simulink model "Test_model"  (R2021a)
settings: Solver=VariableStepAuto  StartTime=0.0  StopTime=5  FixedStep=0.1  RelTol=1e-3
values from neighbouring files (symbols this model uses):
  model = robotics.core.internal.navigation.ModelFactory.getMotionModel(obj.ModelType, obj.DataType)    [StateVector2StructModForEach.m]
  N_j = nonzeros(N_j)    [coordination_linear.m]    (also in init_traj.m = constraints.N_j)
  r = constraints.r    [init_traj.m]
  x0 = constraints.x0    [init_traj.m]
undefined symbols (not defined in the file or in its folder): ADMM_vec, constraints_struct, Objective
libraries: dspswit3 x1, uavGuidanceForEachMod x1, dspindex x1
settings Model: Creator=worc4873  LastModifiedBy=worc4873
settings DebuggingCC: ReadBeforeWriteMsg=DisableAll  WriteAfterWriteMsg=DisableAll  WriteAfterReadMsg=DisableAll  MultiTaskDSMMsg=none
settings ModelReferenceCC: UpdateModelReferenceTargets=IfOutOfDate
settings SFSimCC: SFSimEcho=off

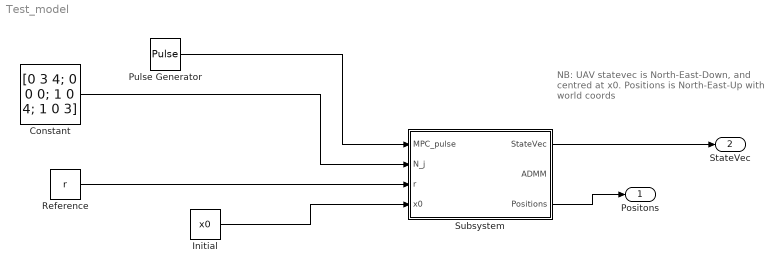
== system Test_model ==
  note: NB: UAV statevec is North-East-Down, and centred at x0. Positions is North-East-Up with world coords
  Constant : Constant  Value=[0 3 4; 0 0 0; 1 0 4; 1 0 3]
  Initial : Constant  Value=x0
  Pulse Generator : DiscretePulseGenerator  Period=10  PhaseDelay=1  SampleTime=0.1
  Reference : Constant  Value=r
  Subsystem : Subsystem
  Positons : Outport
  StateVec : Outport  Port=2
  wires:
  Pulse Generator/1 -> Subsystem/1(MPC_pulse)
  Constant/1 -> Subsystem/2(N_j)
  Reference/1 -> Subsystem/3(r)
  Initial/1 -> Subsystem/4(x0)
  Subsystem/1(StateVec) -> StateVec/1
  Subsystem/3(Positions) -> Positons/1

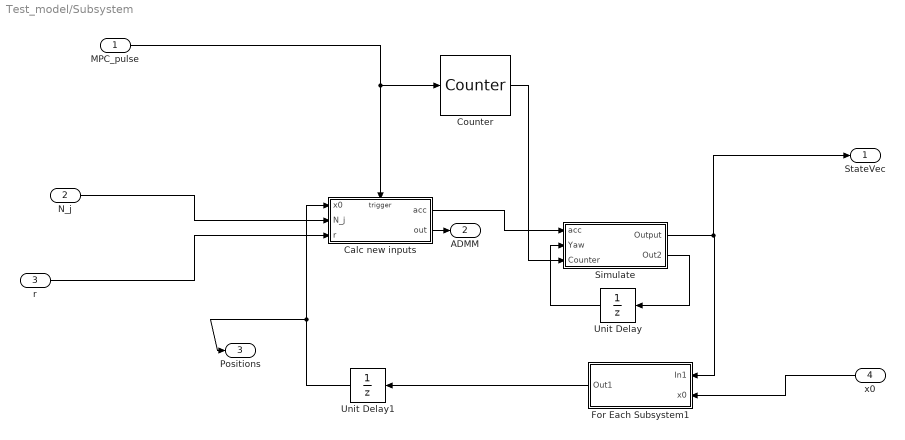
== system Test_model/Subsystem ==
  MPC_pulse : Inport
  N_j : Inport  Port=2
  r : Inport  Port=3
  x0 : Inport  Port=4
  Calc new inputs : Subsystem  TreatAsAtomicUnit=on
  Counter : dspswit3/Counter  Direction=Up  CountEvent=Free running  CounterSize=User defined  MaxCount=30  InitialCount=0  Output=Count  HitValue=32  ResetInput=on  SamplesPerFrame=1  Ts=0.1  CntDtype=double  HitDtype=Logical
  For Each Subsystem1 : Subsystem  TreatAsAtomicUnit=on
  Simulate : Subsystem  TreatAsAtomicUnit=on
  Unit Delay : UnitDelay  SampleTime=-1  HasFrameUpgradeWarning=on
  Unit Delay1 : UnitDelay  InitialCondition=x0  SampleTime=-1  HasFrameUpgradeWarning=on
  StateVec : Outport
  ADMM : Outport  Port=2
  Positions : Outport  Port=3
  wires:
  Unit Delay1/1 -> Positions/1, Calc new inputs/1(x0)
  Simulate/2(Out2) -> Unit Delay/1
  Simulate/1(Output) -> StateVec/1, For Each Subsystem1/1(In1)
  Unit Delay/1 -> Simulate/2(Yaw)
  MPC_pulse/1 -> Counter/1, Calc new inputs/Trigger
  For Each Subsystem1/1(Out1) -> Unit Delay1/1
  Calc new inputs/1(acc) -> Simulate/1(acc)
  Counter/1 -> Simulate/3(Counter)
  Calc new inputs/2(out) -> ADMM/1
  N_j/1 -> Calc new inputs/2(N_j)
  r/1 -> Calc new inputs/3(r)
  x0/1 -> For Each Subsystem1/2(x0)

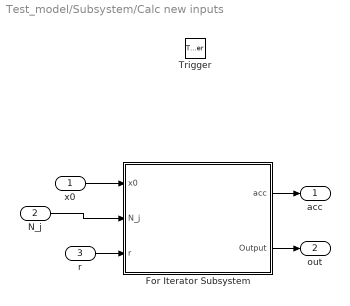
== system Test_model/Subsystem/Calc new inputs ==
  x0 : Inport
  N_j : Inport  Port=2
  r : Inport  Port=3
  Trigger : TriggerPort  VariantControl=(inherit)
  For Iterator Subsystem : Subsystem  TreatAsAtomicUnit=on
  acc : Outport
  out : Outport  Port=2
  wires:
  x0/1 -> For Iterator Subsystem/1(x0)
  N_j/1 -> For Iterator Subsystem/2(N_j)
  r/1 -> For Iterator Subsystem/3(r)
  For Iterator Subsystem/1(acc) -> acc/1
  For Iterator Subsystem/2(Output) -> out/1

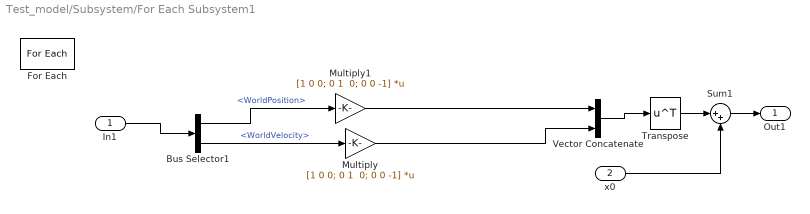
== system Test_model/Subsystem/For Each Subsystem1 ==
  In1 : Inport  Partition=on  PartitionDimension=2  PartitionWidth=1  PartitionOffset=0
  x0 : Inport  Port=2  Partition=on  PartitionDimension=1  PartitionWidth=1  PartitionOffset=0
  Bus Selector1 : BusSelector  OutputSignals=WorldPosition,WorldVelocity
  For Each : ForEach  DisableCoverage=on
  Multiply : Gain  Gain="[1 0 0; 0 1  0; 0 0 -1]"  Multiplication=Matrix(K*u) (u vector)
  Multiply1 : Gain  Gain="[1 0 0; 0 1  0; 0 0 -1]"  Multiplication=Matrix(K*u) (u vector)
  Sum1 : Sum  Inputs=|++
  Transpose : Math  Operator=transpose  SaturateOnIntegerOverflow=on
  Vector Concatenate : Concatenate
  Out1 : Outport  ConcatenationDimension=1
  wires:
  In1/1 -> Bus Selector1/1
  Bus Selector1/2 -> Multiply/1  "<WorldVelocity>"
  Multiply/1 -> Vector Concatenate/2
  Vector Concatenate/1 -> Transpose/1
  Bus Selector1/1 -> Multiply1/1  "<WorldPosition>"
  Multiply1/1 -> Vector Concatenate/1
  x0/1 -> Sum1/2
  Transpose/1 -> Sum1/1
  Sum1/1 -> Out1/1

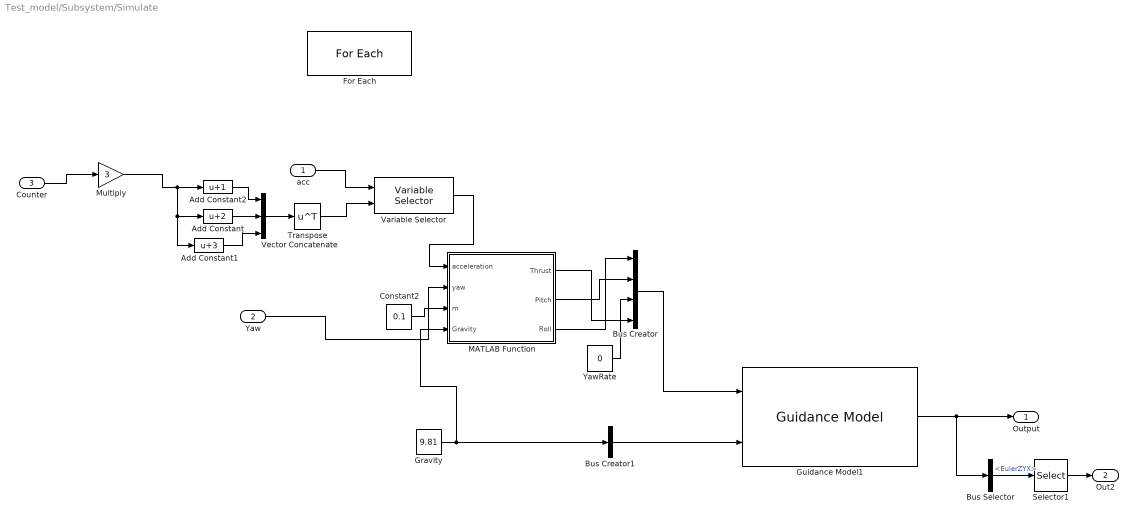
== system Test_model/Subsystem/Simulate ==
  acc : Inport  Partition=on  PartitionDimension=2  PartitionWidth=1  PartitionOffset=0
  Yaw : Inport  Port=2  Partition=on  PartitionDimension=2  PartitionWidth=1  PartitionOffset=0
  Counter : Inport  Port=3
  Add Constant : Bias  Bias=2
  Add Constant1 : Bias  Bias=3
  Add Constant2 : Bias  Bias=1
  Bus Creator : BusCreator  Inputs=4  OutDataTypeStr=Bus: MultirotorGuidanceControlBus  NonVirtualBus=on
      settings: InheritFromInputs=off
  Bus Creator1 : BusCreator  Inputs=1  OutDataTypeStr=Bus: MultirotorGuidanceEnvironmentBus  NonVirtualBus=on
      settings: InheritFromInputs=off
  Bus Selector : BusSelector  OutputSignals=EulerZYX
  Constant2 : Constant  Value=0.1
  For Each : ForEach  DisableCoverage=on
  Gravity : Constant  Value=9.81
  Guidance Model1 : uavGuidanceForEachMod/Guidance Model  ModelType=MultirotorGuidance  SpecifiedDataType=double  SimulateUsing=Code generation  InitialWorldPositionMultirotor=[0; 0; 0]  InitialWorldVelocityMultirotor=[0; 0; 0]  InitialEulerZYXMultirotor=[0; 0; 0]  InitialBodyAngularRateRPYMultirotor=[0; 0; 0]  InitialThrustMultirotor=0  InitialNorthFixedWing=0  InitialEastFixedWing=0  InitialHeightFixedWing=0  InitialAirSpeedFixedWing=0  InitialHeadingAngleFixedWing=0  InitialFlightPathAngleFixedWing=0  InitialRollAngleFixedWing=0  InitialRollAngleRateFixedWing=0  PDRollMultirotor=[3402.97,116.67]  PDPitchMultirotor=[3402.97, 116.67]  PYawRateMultirotor=1950  PThrustMultirotor=3900  MassMultirotor=0.1  PHeightFixedWing=3.9  PHeadingAngleFixedWing=3.9  PFlightPathAngleFixedWing=39  PDRollFixedWing=[3402.97, 116.67]  PAirSpeedFixedWing=1  FlightPathAngleLimitsFixedWing=[-pi/2, pi/2]  StateBusName='MultirotorGuidanceStateBus'  ControlBusName='MultirotorGuidanceControlBus'  EnvironmentBusName='MultirotorGuidanceEnvironmentBus'  DataType=double
  MATLAB Function : MATLAB Function  TreatAsAtomicUnit=on
  Multiply : Gain  Gain=3
  Selector1 : Selector  InputPortWidth=3  IndexOptions=Index vector (dialog)  Indices=1  OutputSizes=1
  Transpose : Math  Operator=transpose  SaturateOnIntegerOverflow=on
  Variable Selector : dspindex/Variable Selector  NumInputs=1  rowsOrCols=Rows  IdxMode=Variable  Elements=[1 3]  ZerOneIdxMode=One-based  errmode=Clip Index  FillMode=on  FillValues=0
  Vector Concatenate : Concatenate  NumInputs=3
  YawRate : Constant  Value=0
  Output : Outport  ConcatenationDimension=2
  Out2 : Outport  Port=2  ConcatenationDimension=2
  wires:
  Guidance Model1/1 -> Bus Selector/1, Output/1
  Bus Creator/1 -> Guidance Model1/1
  MATLAB Function/3(Roll) -> Bus Creator/1
  MATLAB Function/2(Pitch) -> Bus Creator/2
  MATLAB Function/1(Thrust) -> Bus Creator/4
  YawRate/1 -> Bus Creator/3
  acc/1 -> Variable Selector/1
  Constant2/1 -> MATLAB Function/3(m)
  Yaw/1 -> MATLAB Function/2(yaw)
  Bus Creator1/1 -> Guidance Model1/2
  Gravity/1 -> MATLAB Function/4(Gravity), Bus Creator1/1
  Bus Selector/1 -> Selector1/1  "<EulerZYX>"
  Selector1/1 -> Out2/1
  Variable Selector/1 -> MATLAB Function/1(acceleration)
  Add Constant/1 -> Vector Concatenate/2
  Add Constant1/1 -> Vector Concatenate/3
  Add Constant2/1 -> Vector Concatenate/1
  Counter/1 -> Multiply/1
  Multiply/1 -> Add Constant1/1, Add Constant/1, Add Constant2/1
  Vector Concatenate/1 -> Transpose/1
  Transpose/1 -> Variable Selector/2

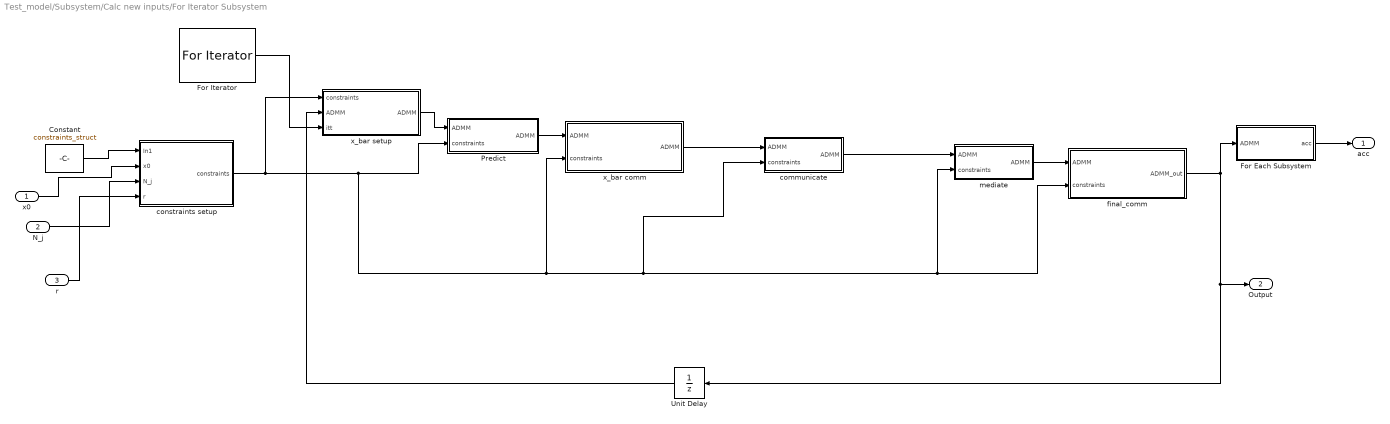
== system Test_model/Subsystem/Calc new inputs/For Iterator Subsystem ==
  x0 : Inport
  N_j : Inport  Port=2
  r : Inport  Port=3
  Constant : Constant  Value=constraints_struct  OutDataTypeStr=Bus: constraints
  For Each Subsystem : Subsystem  TreatAsAtomicUnit=on
  For Iterator : ForIterator  IterationLimit=45
  Predict : Subsystem  TreatAsAtomicUnit=on
  Unit Delay : UnitDelay  InitialCondition=ADMM_vec  SampleTime=-1  HasFrameUpgradeWarning=on
  communicate : Subsystem  TreatAsAtomicUnit=on
  constraints setup : Subsystem  TreatAsAtomicUnit=on
  final_comm : MATLAB Function  TreatAsAtomicUnit=on
  mediate : Subsystem  TreatAsAtomicUnit=on
  x_bar comm : MATLAB Function  TreatAsAtomicUnit=on
  x_bar setup : MATLAB Function  TreatAsAtomicUnit=on
  acc : Outport
  Output : Outport  Port=2
  wires:
  Constant/1 -> constraints setup/1(In1)
  Predict/1(ADMM) -> x_bar comm/1("ADMM ")
  x_bar comm/1(ADMM) -> communicate/1("ADMM ")
  communicate/1(ADMM) -> mediate/1("ADMM ")
  mediate/1(ADMM) -> final_comm/1(ADMM)
  final_comm/1(ADMM_out) -> Output/1, Unit Delay/1, For Each Subsystem/1(ADMM)
  For Each Subsystem/1(acc) -> acc/1
  constraints setup/1(constraints) -> x_bar setup/1(constraints), Predict/2(constraints), x_bar comm/2(constraints), final_comm/2(constraints), mediate/2(constraints), communicate/2(constraints)
  x0/1 -> constraints setup/2(x0)
  N_j/1 -> constraints setup/3(N_j)
  r/1 -> constraints setup/4(r)
  For Iterator/1 -> x_bar setup/3(itt)
  Unit Delay/1 -> x_bar setup/2("ADMM ")
  x_bar setup/1(ADMM) -> Predict/1("ADMM ")

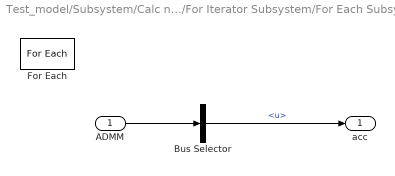
== system Test_model/Subsystem/Calc new inputs/For Iterator Subsystem/For Each Subsystem ==
  ADMM : Inport  Partition=on  PartitionDimension=1  PartitionWidth=1  PartitionOffset=0
  Bus Selector : BusSelector  OutputSignals=u
  For Each : ForEach  DisableCoverage=on
  acc : Outport  ConcatenationDimension=2
  wires:
  ADMM/1 -> Bus Selector/1
  Bus Selector/1 -> acc/1  "<u>"

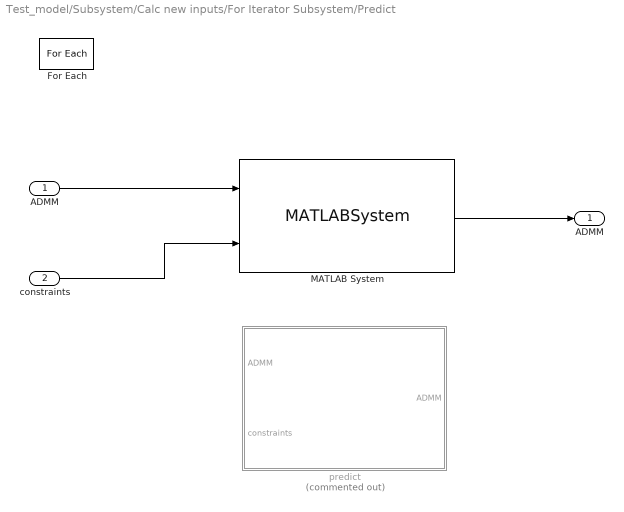
== system Test_model/Subsystem/Calc new inputs/For Iterator Subsystem/Predict ==
  "ADMM " : Inport  OutDataTypeStr=Bus: ADMM  Partition=on  PartitionDimension=1  PartitionWidth=1  PartitionOffset=0
  constraints : Inport  Port=2  OutDataTypeStr=Bus: constraints  Partition=on  PartitionDimension=1  PartitionWidth=1  PartitionOffset=0
  For Each : ForEach  DisableCoverage=on
  MATLAB System : MATLABSystem  System=predictADMM  N=30  delta=0.5  M=4  SampleTime=0.1  OffsetTime=0.05  TickTime=0.1  SimulateUsing=Interpreted execution
      mask Type: predictADMM
      mask Display:
      | disp('predictADMM');
      | port_label('input',1,'ADMM_input');
      | port_label('input',2,'constraints');
      | port_label('output',1,'ADMM_update');
  predict : MATLAB Function  Commented=on  TreatAsAtomicUnit=on
  ADMM : Outport  ConcatenationDimension=1
  wires:
  constraints/1 -> MATLAB System/2
  "ADMM "/1 -> MATLAB System/1
  MATLAB System/1 -> ADMM/1

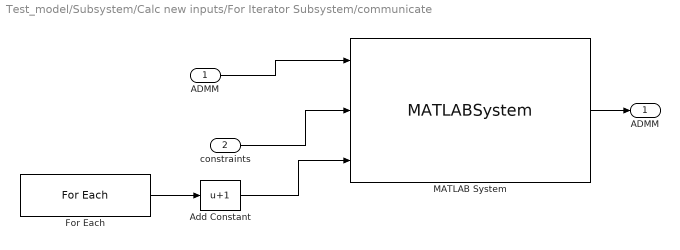
== system Test_model/Subsystem/Calc new inputs/For Iterator Subsystem/communicate ==
  "ADMM " : Inport  OutDataTypeStr=Bus: ADMM  Partition=on  PartitionDimension=1  PartitionWidth=1  PartitionOffset=0
  constraints : Inport  Port=2  OutDataTypeStr=Bus: constraints  Partition=on  PartitionDimension=1  PartitionWidth=1  PartitionOffset=0
  Add Constant : Bias  Bias=1
  For Each : ForEach  DisableCoverage=on  ShowIterationIndex=on
  MATLAB System : MATLABSystem  System=CoordinateADMM  N=30  delta=0.5  M=4  SampleTime=0.1  OffsetTime=0.05  TickTime=0.1  SimulateUsing=Interpreted execution
      mask Type: CoordinateADMM
      mask Display:
      | disp('CoordinateADMM');
      | port_label('input',1,'ADMM_input');
      | port_label('input',2,'constraints');
      | port_label('input',3,'i');
      | port_label('output',1,'ADMM_update');
  ADMM : Outport  ConcatenationDimension=1
  wires:
  "ADMM "/1 -> MATLAB System/1
  constraints/1 -> MATLAB System/2
  MATLAB System/1 -> ADMM/1
  For Each/1 -> Add Constant/1
  Add Constant/1 -> MATLAB System/3

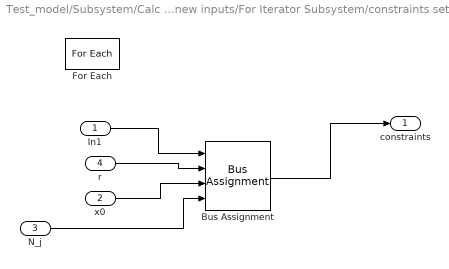
== system Test_model/Subsystem/Calc new inputs/For Iterator Subsystem/constraints setup ==
  In1 : Inport  Partition=on  PartitionDimension=1  PartitionWidth=1  PartitionOffset=0
  x0 : Inport  Port=2  Partition=on  PartitionDimension=1  PartitionWidth=1  PartitionOffset=0
  N_j : Inport  Port=3  Partition=on  PartitionDimension=1  PartitionWidth=1  PartitionOffset=0
  r : Inport  Port=4  Partition=on  PartitionDimension=1  PartitionWidth=1  PartitionOffset=0
  Bus Assignment : BusAssignment  AssignedSignals=r,x0,N_j
  For Each : ForEach  DisableCoverage=on
  constraints : Outport  ConcatenationDimension=1
  wires:
  In1/1 -> Bus Assignment/1
  Bus Assignment/1 -> constraints/1
  r/1 -> Bus Assignment/2
  x0/1 -> Bus Assignment/3
  N_j/1 -> Bus Assignment/4

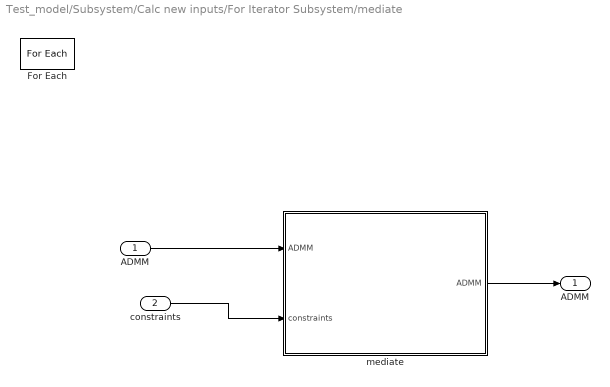
== system Test_model/Subsystem/Calc new inputs/For Iterator Subsystem/mediate ==
  "ADMM " : Inport  Partition=on  PartitionDimension=1  PartitionWidth=1  PartitionOffset=0
  constraints : Inport  Port=2  Partition=on  PartitionDimension=1  PartitionWidth=1  PartitionOffset=0
  For Each : ForEach  DisableCoverage=on
  mediate : MATLAB Function  TreatAsAtomicUnit=on
  ADMM : Outport  ConcatenationDimension=1
  wires:
  "ADMM "/1 -> mediate/1("ADMM ")
  constraints/1 -> mediate/2(constraints)
  mediate/1(ADMM) -> ADMM/1

== matlab function Test_model/Subsystem/Calc new inputs/For Iterator Subsystem/Predict/predict ==
  data: ADMM input Bus: ADMM; ADMM output; Objective parameter; model parameter; constraints input Bus: constraints
function ADMM = predict_step(ADMM,Objective, model, constraints)

Q = Objective.Q;
R = Objective.R;
N = Objective.N;

Nd = 3;
nx = size(Q,1);
nu = size(R,1);

A = model.A;
B = model.B;
umax = model.umax;
umin = model.umin;


N_j = constraints.N_j;
r = constraints.r;
x0 = constraints.x0;

rho = ADMM.rho;
lambda = ADMM.lambda;
lambda_from_j = ADMM.lambda_from_j;
w = ADMM.w;
w_from_j = ADMM.w_from_j;

min_input = repmat(ones(nu,1)*umin,N,1);
max_input = repmat(ones(nu,1)*umax,N,1);
% - linear dynamics

u_bound = [inf((N+1)*nx,1);max_input];
l_bound = [-inf((N+1)*nx,1);min_input];


posM = blkdiag(eye(Nd),zeros(nx-Nd)); % Matrix to take only position from the state vector x (zeros rest)
d = [eye(Nd),zeros(Nd,nx-Nd)]; % Matrix to take only position from the state vector x (only returns pos)
posMN = kron(eye(N+1),d); %returns pos across time steps

Ax = kron(speye(N+1), -speye(nx)) + kron(sparse(diag(ones(N, 1), -1)), A);
Bu = kron([sparse(1, N); speye(N)], B);
Aeq = [Ax, Bu];
b_eq = [-x0'; zeros(N*nx, 1)];
P_new = blkdiag( kron(eye(N), Q+ (size(N_j,2)+1)*rho/2*posM ), Q+(size(N_j,2)+1)*rho/2*posM, kron(eye(N), R) );

q = prediction_linear(lambda,lambda_from_j,w,w_from_j,rho,r',Q,N,nu,posMN);

qp_opts = optimoptions('quadprog','Display','off','Algorithm','active-set');
init = [ADMM.x;ADMM.u];
res = quadprog(P_new,q,[],[], full(Aeq),b_eq,l_bound,u_bound,init,qp_opts);
ADMM.x = res(1:nx*(N+1));
ADMM.u = res((N+1)*nx+1:end);

end

== matlab function Test_model/Subsystem/Calc new inputs/For Iterator Subsystem/x_bar comm ==
  data: ADMM input Bus: ADMM; ADMM output; constraints input Bus: constraints
function ADMM = comm_xbar(ADMM,constraints)

for i =1:size(ADMM,1)
    ADMM(i).x_bar(:,i) = ADMM(i).x;
    nonzero_N_j = nonzeros(constraints(i).N_j);
    for j = 1:nnz(constraints(i).N_j)
        ADMM(i).x_bar(:,nonzero_N_j(j)) = ADMM(nonzero_N_j(j)).x;
    end
end

end

== matlab function Test_model/Subsystem/Calc new inputs/For Iterator Subsystem/final_comm ==
  data: ADMM input Bus: ADMM; ADMM_out output Bus: ADMM size=4 1; constraints input Bus: constraints
function ADMM_out = final_comm(ADMM,constraints)
    
ADMM_out = ADMM;
    for i = 1:size(ADMM_out,1)
        nonzero_N_j = nonzeros(constraints(i).N_j);
        for j = 1:nnz(constraints(i).N_j)
            curr_comm = nonzero_N_j(j);
            ADMM_out(i).lambda_from_j(:,nonzero_N_j(j)) = ADMM_out(curr_comm).lambda_to_j(:,i);
            ADMM_out(i).w_from_j(:,nonzero_N_j(j)) = ADMM_out(curr_comm).w_to_j(:,i);
        end
        
    end
    
end

== matlab function Test_model/Subsystem/Calc new inputs/For Iterator Subsystem/mediate/mediate ==
  data: ADMM input Bus: ADMM; ADMM output; N parameter; constraints input Bus: constraints
function ADMM = mediate_step(ADMM,N, constraints)

Nd = 3;
nx = size(ADMM.x,1)/(N+1);

d = [eye(Nd),zeros(Nd,nx-Nd)]; % Matrix to take only position from the state vector x (only returns pos)
posMN = kron(eye(N+1),d); %returns pos across time steps


ADMM.lambda = ADMM.lambda + ADMM.rho * (posMN * ADMM.x-ADMM.w);
nonzero_N_j = nonzeros(constraints.N_j);
for j = 1:nnz(constraints.N_j)
    ADMM.lambda_to_j(:,nonzero_N_j(j)) = ADMM.lambda_to_j(:,nonzero_N_j(j)) + ADMM.rho * (posMN*ADMM.x_bar(:,nonzero_N_j(j)) - ADMM.w_to_j(:,nonzero_N_j(j)));
end

end

== matlab function Test_model/Subsystem/Simulate/MATLAB Function ==
  data: acceleration input; Thrust output; yaw input; m input; Pitch output; Roll output; Gravity input
function [Thrust,Pitch,Roll] = acc_to_input(acceleration,yaw,m,Gravity)

 
    Pitch = atan2((-acceleration(1)*cos(yaw)-acceleration(2)*sin(yaw)), (acceleration(3) + Gravity));
    Roll = atan2(((-acceleration(1)*sin(yaw)+acceleration(2)*cos(yaw))*cos(Pitch)), (acceleration(3)+Gravity));
    
    Thrust = m*(acceleration(3)+Gravity)/(cos(Pitch)*cos(Roll));

end

== matlab function Test_model/Subsystem/Calc new inputs/For Iterator Subsystem/x_bar setup ==
  data: constraints input Bus: constraints; ADMM output; ADMM input Bus: ADMM; Objective parameter; model parameter; itt input
function ADMM = fcn(constraints,ADMM,Objective, model, itt)

if itt == 1
    nx = size(Objective.Q,2);
    nu = size(Objective.R,1);
    N = Objective.N;
    M = size(ADMM,1);
    
    x_init = zeros(nx*(N+1),M);
    u_init = zeros(nu*N,M);
    for i = 1:M
%         Ax = kron(speye(N+1), -speye(nx)) + kron(sparse(diag(ones(N, 1), -1)), model.A);
%         Bu = kron([sparse(1, N); speye(N)], model.B);
%         b_eq = [-constraints(i).x0 zeros(1, N*nx)]';
        [x_init(:,i),u_init(:,i)] = init_traj(ADMM(i).rho,Objective,constraints(i),model); %initial solution
%         init_vel = constraints(i).x0(4:6)';
%         T = model.B(4,1);
%         steps = round(max(abs(init_vel))/(T*model.umax));
%         steps = min(steps,N);
%         if steps >= 1
%             u_start = model.umax/max(abs(init_vel))*-init_vel;
%             final_vel = init_vel + T*(steps-1)*u_start;
%             u_start = repmat(u_start,steps-1,1);
%             u_start = [u_start;-final_vel/T];
%         else
%             u_start = [];
%         end
%         u_init(:,i) = [u_start;zeros(N*nu-size(u_start,1),1)];
%         x_init(:,i) = (Ax)\(b_eq - Bu*u_init(:,i));
%         direction = constraints(i).r(1:3)'-x_init(nx*N+1:nx*N+3,i);
%         start = floor((N-size(u_start,1)/nu)/2);
%         for k = 1:100
%             
%             accel = (model.umax/max(abs(direction)))*direction;
%             u_init(steps*nu+1:(steps+start)*nu,i) = repmat(accel,start,1);
%             if steps+2*start < N
%                 u_init((steps+start)*nu+1:(steps+2*start)*nu,i) = -repmat(accel,start,1);
%             else
%                 u_init((steps+start)*nu+1:end,i) = -repmat(accel, N-steps-start,1);
%             end
%             x_init(:,i) = (Ax)\(b_eq - Bu*u_init(:,i));
%             
%             final_diff = constraints(i).r(1:3)'-x_init(nx*N+1:nx*N+3,i);
%             final_diff = final_diff';
%             
%             if norm(x_init(nx*N+1:end,i)-constraints(i).r') < 0.1
%                 break;
%             elseif sign(dot(final_diff,direction)) ~= 1
%                 start = start - 1;
%                 u_init(:,i) = [u_start;zeros(N*nu-size(u_start,1),1)];
%                 x_init(:,i) = (Ax)\(b_eq - Bu*u_init(:,i));
%             else
%                 break;
%             end
%         end
        %accel in direction of target, then max deccel, start deccel at N/2
        %and tune from there
    end
    for i =1:M
        ADMM(i).x = x_init(:,i);
        ADMM(i).u = u_init(:,i);
        ADMM(i).x_bar(:,i) = x_init(:,i);
        nonzero_N_j = nonzeros(constraints(i).N_j);
        for j = 1:nnz(constraints(i).N_j)
            ADMM(i).x_bar(:,nonzero_N_j(j)) = x_init(:,nonzero_N_j(j));
        end
    end
end

end
